simulink model "missile_ADRC_full"  (R2025b)
settings: Solver=VariableStepAuto  StartTime=0.0  StopTime=40  RelTol=1e-3
settings Model: Creator=91872  LastModifiedBy=91872

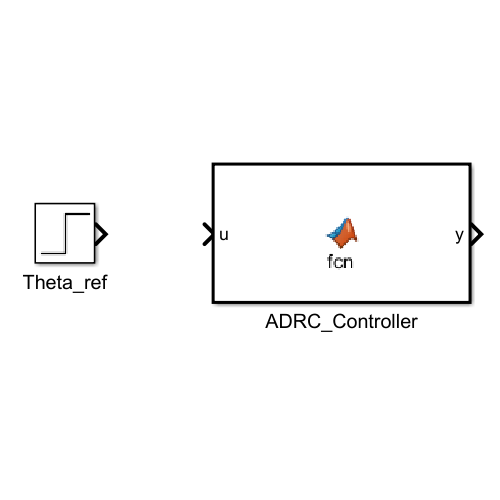
[thumbnail: Simulink's stored preview of the top-level diagram]
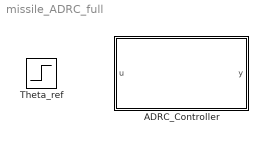
== system missile_ADRC_full ==
  ADRC_Controller : MATLAB Function  TreatAsAtomicUnit=on
  Theta_ref : Step  After=5*pi/180  SampleTime=0

== matlab function missile_ADRC_full/ADRC_Controller ==
  data: u input; y output
function y = fcn(u)

y = u;
